simulink model "SimulinkPinson"  (R2019b)
settings: Solver=VariableStepAuto  StartTime=0.0  StopTime=6031  RelTol=1e-3
libraries: simulink x1
settings Model: Creator=pieterpinson  LastModifiedBy=pieterpinson

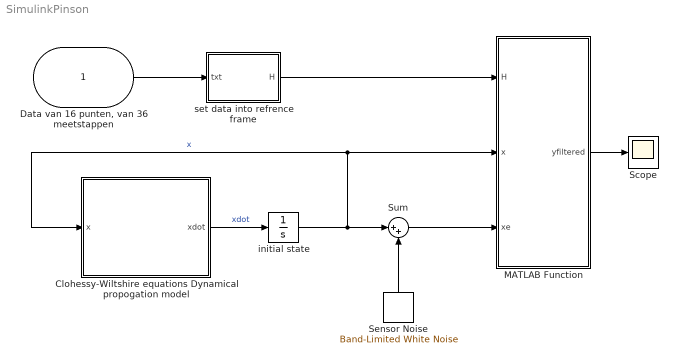
== system SimulinkPinson ==
  "Data van 16 punten, van 36 meetstappen" : Inport
  Clohessy-Wiltshire equations Dynamical propogation model : MATLAB Function  TreatAsAtomicUnit=on
  MATLAB Function : MATLAB Function  TreatAsAtomicUnit=on
  Scope : Scope
  Sensor Noise : simulink/Sources/Band-Limited White Noise  Cov=[0.1]  Ts=0.1  seed=[23341]
  Sum : Sum  Inputs=|++
  initial state : Integrator  InitialCondition=|
      | [-2.9671 ; 0.5236
      | ; -1.3963 ; -0.0873 ; -0.1489 ; 0.0262]
  set data into refrence frame : MATLAB Function  TreatAsAtomicUnit=on
  wires:
  "Data van 16 punten, van 36 meetstappen"/1 -> set data into refrence frame/1(txt)
  Clohessy-Wiltshire equations Dynamical propogation model/1(xdot) -> initial state/1  "xdot"
  initial state/1 -> Clohessy-Wiltshire equations Dynamical propogation model/1(x), MATLAB Function/2(x), Sum/1  "x"
  Sensor Noise/1 -> Sum/2
  MATLAB Function/1(yfiltered) -> Scope/1
  set data into refrence frame/1(H) -> MATLAB Function/1(H)
  Sum/1 -> MATLAB Function/3(xe)

== matlab function SimulinkPinson/set data into refrence frame ==
  data: txt input; H output
function H = measurements(txt)

    H = 239/txt;
end

== matlab function SimulinkPinson/Clohessy-Wiltshire equations Dynamical propogation model ==
  data: x input; xdot output
function xdot = SCmodel(x)

Q = 10^-6*[1 ;1 ;1];

thetadot = A*x;
omegadot = Omega*P*omega + Q;

xdot = [thetadot omegadot];

end

== matlab function SimulinkPinson/MATLAB Function ==
  data: H input; x input; xe input; yfiltered output
function yfiltered = Kalmanfilter(H,x,xe)

    K = 0.1*[1 ; 1 ; 1];%kalman gain
    
    xe = sensored;
    
    yfiltered = x + K*(xe-H);
    
end
